simulink model "LateralControl_PI_P"  (R2021b)
settings: Solver=VariableStepAuto  StartTime=0.0  StopTime=112  RelTol=1e-3
InitFcn:
  | clear all;
  | 
  | 
  | %Path in global coordinate reference frame - X and Y
  | 
  | xRef=[57.22167206
  | 52.70709991
  | 48.87397385
  | 44.3594017
  | 39.93001175
  | 35.15989685
  | 31.07122803
  | 16.59052467
  | 7.391020298
  | -2.57510972
  | -9.900641441
  | -13.56340694
  | -16.28918648
  | -17.56689644
  | -15.43738079
  | -8.537752151
  | -2.745471001
  | 1.002475381
  | 6.624394894
  | 10.62788296
  | 15.6535387
  | 20.93473625
  | 24.85304451
  | 28.26026726
  | 31.32676888
  | 33.79700851
  | 35.84134293
  | 36.18206406
  | 35.67097855
  | 34.47845078
  | 32.00821304
  | 29.96388054
  | 28.00472641
  | 26.30111313
  | 25.10858536
  | 24.00123787
  | 23.14943123
  | 22.38280678
  | 21.95690346
  | 21.53100014
  | 21.1902771
  | 20.84955597
  | 20.59401321
  | 21.10509682
  | 21.53100014
  | 21.7013607
  | 21.7013607
  | 21.53100014
  | 21.36063957
  | 21.44581985
  | 22.04208374
  | 23.8308773
  | 25.87521172
  | 28.77135086
  | 35.24507523
  | ... (+152 lines)
libraries: autolibutils x4, slpidlib x3, autolibshared x2, vehdynlibviscommon x1, simulink x1, sim3dlib x1, vdynlib x1, vehdynlibsteering x1, eeGeneralControl x1
(part 3 of 3)

== matlab function LateralControl_PI_P/MATLAB Function1 ==
  data: xRef input; yRef input; yawRef input; x_actual input; y_actual input; pose input; psi_error output; lat_dev output
function [psi_error, lat_dev]    = compute(xRef, yRef,yawRef, x_actual, y_actual, pose)

x_shifted=xRef-x_actual;
y_shifted=yRef-y_actual;

deg=360-((180/3.14)*pose);
matrix=[cosd(deg) -sind(deg);
        sind(deg) cosd(deg)];
K=cat(2,x_shifted,y_shifted);
K=K';
transformed=matrix*K;
x_path=transformed(1,:)-1.135;
y_path=transformed(2,:);
yaw_path=yawRef-pose;

distance_nearest = ((x_path.^2) +(y_path.^2)).^(0.5);
[~, index_nearest] = min(distance_nearest);
psi_error=yaw_path(index_nearest);
lat_dev=y_path(index_nearest);
end

== matlab function LateralControl_PI_P/Path_smoothing_function ==
  data: u1 input; xRef output; u2 input; yRef output; yawRef output
function [xRef,yRef,yawRef] = fcn(u1,u2)

yaw=zeros(size(u1));
directionRef=ones(size(u1));
refPoses=[u1 u2 yaw];
refDirections=[directionRef];
numSmoothPoses=4500;
[poses,~] = smoothPathSpline(refPoses,refDirections,numSmoothPoses);

xRef=poses(:,1);
yRef=poses(:,2);
yawRef=poses(:,3);
yawRef=unwrap(pi*yawRef/180);

end
